simulink model "COMP_ELEC"  (R2026b)
settings: Solver=VariableStepAuto
undefined symbols (not defined in the file or in its folder): Ke
libraries: fl_lib x9, ee_lib x3, nesl_utility x3, simulink x1
settings Model: Creator=bhorton  LastModifiedBy=bhorton

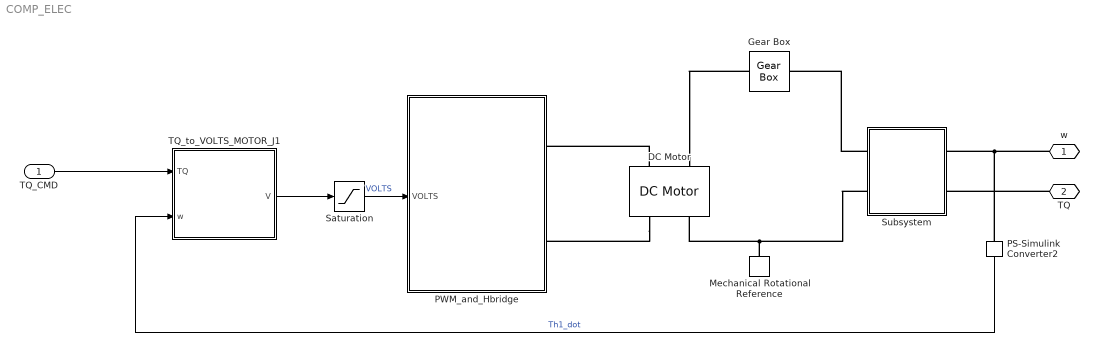
== system COMP_ELEC ==
  TQ_CMD : Inport
  DC Motor : ee_lib/Electromechanical/Brushed Motors/DC Motor  PartSpecification="{\"CollectionId\":\"MW.SimscapeElectrical\",\"CollectionVersion\":\"1.0.0\",\"DatasetId\":\"Maxon|RE_65_388985_24|simscape.electrical.dcMotor\",\"DisplayName\":\"Maxon:RE_65_388985_24\"}"  field_option=ee.enum.field_option.pm  Rf=100 % Parameter not set Ohm  Lf=1 % Parameter not set H  Laf=0.15 % Parameter not set H  If0=0 % Parameter not set A  parameterization=ee.enum.dcparam_option.circuit_param  Ra=0.0891 % Datasheet derived Ohm  La=0.031 % Datasheet derived mH  emf_or_torque=ee.enum.emf_or_torque.ki  Kv=5.62345 % Parameter estimated mV/rpm  Ki=53.7 % Datasheet derived mN*m/A  T_stall=0.24e-3 % Parameter not set N*m  w_max=19100 % Parameter not set rpm  w_rated=15000 % Parameter not set rpm  P_rated=0.08 % Parameter not set W  V_rated=1.5 % Parameter not set V  lam_param=ee.enum.lam_param.current  i_noload=0.697 % Datasheet derived A  V_i_noload=24 % Datasheet derived V  J=1290 % Datasheet derived g*cm^2  lam=0 % % Parameter not set mN*m/(rad/s)  speed0=0 % Parameter not set rpm  alpha=3.93e-3 % Parameter not set 1/K  Tmeas=25 % Parameter not set degC  thermal_mass=667.588357588358 % Parameter estimated J/K  initial_temperature=25 % Parameter not set degC
      settings: AttributesFormatString=Maxon:RE_65_388985_24
  Gear Box : fl_lib/Mechanical/Mechanisms/Gear Box  ratio=25  t_in_specify=off  t_in_priority=None  t_in=0 N*m  t_in_nominal_specify=off  t_in_nominal_value=1  t_in_nominal_unit=N*m  t_out_specify=off  t_out_priority=None  t_out=0 N*m  t_out_nominal_specify=off  t_out_nominal_value=1  t_out_nominal_unit=N*m
      settings: AttributesFormatString=|
      | GEAR_RATIO = w_in/w_out
      | GEAR_RATIO =  %<ratio>
  Mechanical Rotational Reference : fl_lib/Mechanical/Rotational Elements/Mechanical Rotational Reference
  PS-Simulink Converter2 : nesl_utility/PS-Simulink Converter  PhysicalDomain=network_engine_domain  SubClassName=ps_output  LeftPortType=input  RightPortType=output  PseudoPeriodic=off  Frequencies=[]  VectorFormat=inherit  Unit=rad/s  AffineConversion=off
  PWM_and_Hbridge : Subsystem
  Saturation : Saturate  UpperLimit=24  LowerLimit=-24
  Subsystem : Subsystem
  TQ_to_VOLTS_MOTOR_J1 : Subsystem  mask(DC motor (w_IN and TQ_out)){R=0.0891, K=53.7/1000, Kb=Ke, b=0.005}
      mask prompts: R "Armature resistance (ohms)"; K "Torque constant (N.m/A)"; Kb "Back Emf constant (V.sec/rad)"; b "damping value (N.m.sec/rad)"
      mask help: A DC motor model that outputs required VOLTAGE needed to deliver a specified TORQUE
      mask DialogControl Control2 Prompt: NOTE:  with SI units, the Toque constant (Ka) and Back EMF constant(Kb) are the same.
      mask DialogControl Container9 Prompt: Electrical
      mask Display: fprintf('DC motor\n(TQ_IN \n and \n V_out)');
  w : PMIOPort  Side=Right
  TQ : PMIOPort  Port=2  Side=Right
  wires:
  PS-Simulink Converter2/1 -> TQ_to_VOLTS_MOTOR_J1/2(w)  "Th1_dot"
  TQ_to_VOLTS_MOTOR_J1/1(V) -> Saturation/1
  Saturation/1 -> PWM_and_Hbridge/1(VOLTS)  "VOLTS"
  TQ_CMD/1 -> TQ_to_VOLTS_MOTOR_J1/1(TQ)
  connections:
  PS-Simulink Converter2/LConn1 -- w/RConn1 -- Subsystem/RConn1
  Subsystem/LConn2 -- DC Motor/RConn2 -- Mechanical Rotational Reference/LConn1
  DC Motor/RConn1 -- PWM_and_Hbridge/RConn2
  DC Motor/LConn1 -- PWM_and_Hbridge/RConn1
  Subsystem/LConn1 -- Gear Box/RConn1
  Gear Box/LConn1 -- DC Motor/LConn2
  TQ/RConn1 -- Subsystem/RConn2

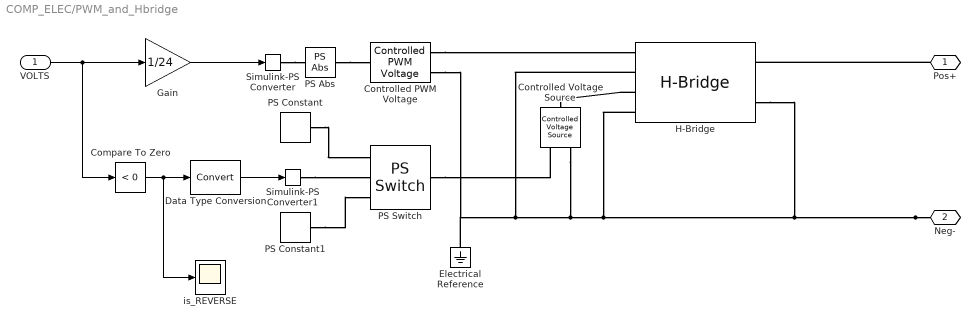
== system COMP_ELEC/PWM_and_Hbridge ==
  VOLTS : Inport
  Compare To Zero : simulink/Logic and Bit Operations/Compare To Zero  relop=<  OutDataTypeStr=uint8
  Controlled PWM Voltage : ee_lib/Integrated Circuits/Controlled PWM Voltage  F=80 kHz  TD=0 s  pulse_width_offset=0 s  pulse_min=0 s  pwm_or_av=ee.enum.pwm_or_av.averaged  event_type=ee.enum.ic.event.asynchronous  sample_time=1e-6 s  Vmin=0 V  Vmax=24 V  Vm=24 V  u_min=0  u_max=1
  Controlled Voltage Source : fl_lib/Electrical/Electrical Sources/Controlled Voltage Source
  Data Type Conversion : DataTypeConversion  SaturateOnIntegerOverflow=off  RndMeth=Floor
  Electrical Reference : fl_lib/Electrical/Electrical Elements/Electrical Reference
  Gain : Gain  Gain=1/24
  H-Bridge : ee_lib/Semiconductors & Converters/Converters/H-Bridge  supply_ports=ee.enum.supply_ports.hidesupply  pwm_or_av=ee.enum.pwm_or_av.averaged  discontinuous=ee.enum.current_profile.continuous  freewheeling_mode=ee.enum.converters.freewheeling_mode.one_switch_one_diode  Rload=10 Ohm  Lload=1e-5 H  F=10 kHz  regenerative_braking_mode=ee.enum.converters.regenerative_braking_mode.always_enabled  Venable=0.1 V  Vmax=24 V  Vreverse=2.5 V  Vbrake=2.5 V  Vm=24 V  Ron=0.1 Ohm  Don=0.05 Ohm  Goff=1e-6 S  Tmeas=298.15 K  Ron2=0.1 Ohm  Don2=0.05 Ohm  Tmeas2=398.15 K  thermal_mass=100 J/K  initial_temperature=298.15 K
  PS Abs : fl_lib/Physical Signals/Nonlinear Operators/PS Abs  ZeroCross=true
  PS Constant : fl_lib/Physical Signals/Sources/PS Constant  constant=5 V
  PS Constant1 : fl_lib/Physical Signals/Sources/PS Constant  constant=0 V
  PS Switch : fl_lib/Physical Signals/Nonlinear Operators/PS Switch  Threshold=0.5  ZeroCross=true
  Simulink-PS Converter : nesl_utility/Simulink-PS Converter  PhysicalDomain=network_engine_domain  SubClassName=ps_input  LeftPortType=input  RightPortType=output  PseudoPeriodic=off  Frequencies=[]  NoiseDistribution=none  NoiseParameters=[]  Unit=1  AffineConversion=off  FilteringAndDerivatives=provide  SimscapeFilterOrder=1  InputFilterTimeConstant=0.001  UdotUserProvided=0
  Simulink-PS Converter1 : nesl_utility/Simulink-PS Converter  PhysicalDomain=network_engine_domain  SubClassName=ps_input  LeftPortType=input  RightPortType=output  PseudoPeriodic=off  Frequencies=[]  NoiseDistribution=none  NoiseParameters=[]  Unit=1  AffineConversion=off  FilteringAndDerivatives=provide  SimscapeFilterOrder=1  InputFilterTimeConstant=0.001  UdotUserProvided=0
  is_REVERSE : Scope
      settings: ActiveDisplayYMinimum=-0.21102162286492421  ActiveDisplayYMaximum=1.2157883377749992  DataLoggingVariableName=ScopeData2
  Pos+ : PMIOPort  Side=Right
  Neg- : PMIOPort  Port=2  Side=Right
  wires:
  Gain/1 -> Simulink-PS Converter/1
  Compare To Zero/1 -> Data Type Conversion/1, is_REVERSE/1
  Data Type Conversion/1 -> Simulink-PS Converter1/1
  VOLTS/1 -> Compare To Zero/1, Gain/1
  connections:
  Simulink-PS Converter1/RConn1 -- PS Switch/LConn2
  H-Bridge/LConn3 -- Controlled Voltage Source/LConn1
  Simulink-PS Converter/RConn1 -- PS Abs/LConn1
  PS Constant1/RConn1 -- PS Switch/LConn3
  PS Constant/RConn1 -- PS Switch/LConn1
  PS Abs/RConn1 -- Controlled PWM Voltage/LConn1
  PS Switch/RConn1 -- Controlled Voltage Source/RConn1
  Neg-/RConn1 -- H-Bridge/RConn2 -- H-Bridge/LConn4 -- Controlled Voltage Source/RConn2 -- H-Bridge/LConn2 -- Electrical Reference/LConn1 -- Controlled PWM Voltage/RConn2
  Controlled PWM Voltage/RConn1 -- H-Bridge/LConn1
  Pos+/RConn1 -- H-Bridge/RConn1

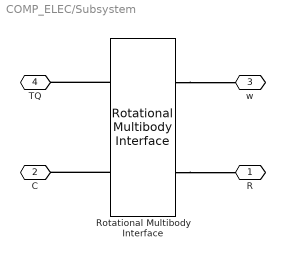
== system COMP_ELEC/Subsystem ==
  Rotational Multibody Interface : fl_lib/Mechanical/Multibody Interfaces/Rotational Multibody Interface
  R : PMIOPort  Side=Left
  C : PMIOPort  Port=2  Side=Left
  w : PMIOPort  Port=3  Side=Right
  TQ : PMIOPort  Port=4  Side=Right
  connections:
  Rotational Multibody Interface/RConn2 -- R/RConn1
  Rotational Multibody Interface/RConn1 -- w/RConn1
  Rotational Multibody Interface/LConn2 -- C/RConn1
  Rotational Multibody Interface/LConn1 -- TQ/RConn1

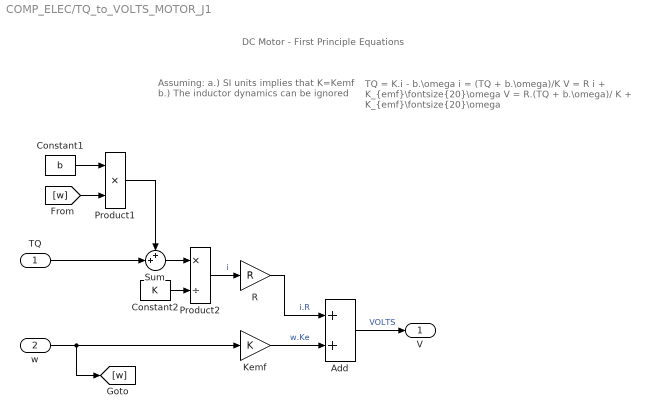
== system COMP_ELEC/TQ_to_VOLTS_MOTOR_J1 ==
  note: Assuming:
      |  a.) SI units implies that   K=Kemf
      |  b.) The inductor dynamics can be ignored
  note: DC Motor - First Principle Equations
  note: TQ = K.i  - b.\omega
      |
      | i = (TQ + b.\omega)/K
      |
      | V = R i   +   K_{emf}\fontsize{20}\omega
      |
      | V = R.(TQ  + b.\omega)/ K   +    K_{emf}\fontsize{20}\omega
  TQ : Inport
  w : Inport  Port=2
  Add : Sum
  Constant1 : Constant  Value=b
  Constant2 : Constant  Value=K
  Kemf : Gain  Gain=K
  Product1 : Product
  Product2 : Product  Inputs=*/
  R : Gain  Gain=R
  Sum : Sum  Inputs=++|
  V : Outport
  wires:
  Product1/1 -> Sum/1
  [w] -> Product1/2
  Constant1/1 -> Product1/1
  TQ/1 -> Sum/2
  Sum/1 -> Product2/1
  Add/1 -> V/1  "VOLTS"
  w/1 -> Kemf/1, [w]
  Kemf/1 -> Add/2  "w.Ke"
  Constant2/1 -> Product2/2
  Product2/1 -> R/1  "i"
  R/1 -> Add/1  "i.R"
